simulink model "gtm_aeromodel"  (Simulink 7.2)
settings: Solver=ode45  StartTime=0.0  StopTime=10.0  RelTol=1e-3
undefined symbols (not defined in the file or in its folder): A_BLCG, A_BW, A_CW, A_FSCG, A_FSREF_in, A_SW, A_WLCG, A_WLREF, ALPHA0, bclowb, bclowbx_FMACH, bcmowb, bcmowbx_FHP, bcmowby_FMACH, cda, cdax_FLPDEF, cddr, cddrx_FMACH, cdo, cdox_FLPDEF, cdt1, cdt1x_mach, cdt2, cdt2x_mach, cdto, cdtox_mach, cdwb, cdwbx_FALPHA, cdwby_FMACH, clat, clatfr, clatfrx_FHP, clatfry_FMACH, clatx_mach, clawbfr, clawbfrx_FHP, clawbfry_FMACH, cldefr, cldefrx_FHP, cldefry_FMACH, cldtab, cldtabx_FMACH, clqwb, clqwbfr, clqwbfrx_FHP, clqwbfry_FMACH, clqwbx_mach, cltdd, cltddx_FHP, cltddy_FMACH, clwb, clwbtdd, clwbtddx_FHP, clwbtddy_FMACH, clwbx_FALPHA, clwby_FMACH, clwbzdd, clwbzddx_FHP, clwbzddy_FMACH, clzdd ... (+196)
libraries: model_lib x1
(part 7 of 10)

== system gtm_aeromodel/get aero forces and moments/AERODYNAMICS/Aero Incidence Angles/DOWNWASH/epswb_plus_alphadot/despoflex ==
  altitude : Inport  OutDataType=sfix(16)  OutScaling=2^0
  Mach : Inport  Port=2  OutDataType=sfix(16)  OutScaling=2^0
  Enable : EnablePort
  Fcn : Fcn  Expr=1/u
  Product : Product  OutDataType=sfix(16)  OutScaling=2^0  SaturateOnIntegerOverflow=on  RndMeth=Zero  InputSameDT=on  OutDataTypeStr=Inherit: Same as first input
  clatfr : Subsystem  mask(2-D Table){y=clatfrx_FHP, z=clatfry_FMACH, tab=clatfr}
      mask prompts: y "Y vector:"; z "Z vector:"; tab "Table:"
      mask help: 2-D Table Look Up. Enter monotonic Y and Z vectors and a matrix of 2-D tables. See the help for more info.
      mask Help: The Y and Z vectors must be monotonic.  Y  indexes into the columns of the 2-D table & Z indexes into the rows of the 2-D tables.   The input values are y and z respectively (e.g., top port = y).
      mask Display: plot(-10,-10,110,110,[90,50,10],[90,40,30],[90,50,10],[50,26,20],[90,50,10],[22,13,10])
  cmatfr : Subsystem  mask(2-D Table){y=cmatfrx_FHP, z=cmatfry_FMACH, tab=cmatfr}
      mask prompts: y "Y vector:"; z "Z vector:"; tab "Table:"
      mask help: 2-D Table Look Up. Enter monotonic Y and Z vectors and a matrix of 2-D tables. See the help for more info.
      mask Help: The Y and Z vectors must be monotonic.  Y  indexes into the columns of the 2-D table & Z indexes into the rows of the 2-D tables.   The input values are y and z respectively (e.g., top port = y).
      mask Display: plot(-10,-10,110,110,[90,50,10],[90,40,30],[90,50,10],[50,26,20],[90,50,10],[22,13,10])
  depsoflex : Subsystem  mask(2-D Table){y=depsoflexx_FHP, z=depsoflexy_FMACH, tab=depsoflex}
      mask prompts: y "Y vector:"; z "Z vector:"; tab "Table:"
      mask help: 2-D Table Look Up. Enter monotonic Y and Z vectors and a matrix of 2-D tables. See the help for more info.
      mask Help: The Y and Z vectors must be monotonic.  Y  indexes into the columns of the 2-D table & Z indexes into the rows of the 2-D tables.   The input values are y and z respectively (e.g., top port = y).
      mask Display: plot(-10,-10,110,110,[90,50,10],[90,40,30],[90,50,10],[50,26,20],[90,50,10],[22,13,10])
  epsafr_ : Subsystem  mask(2-D Table){y=epsafrx_FHP, z=epsafry_FMACH, tab=epsafr}
      mask prompts: y "Y vector:"; z "Z vector:"; tab "Table:"
      mask help: 2-D Table Look Up. Enter monotonic Y and Z vectors and a matrix of 2-D tables. See the help for more info.
      mask Help: The Y and Z vectors must be monotonic.  Y  indexes into the columns of the 2-D table & Z indexes into the rows of the 2-D tables.   The input values are y and z respectively (e.g., top port = y).
      mask Display: plot(-10,-10,110,110,[90,50,10],[90,40,30],[90,50,10],[50,26,20],[90,50,10],[22,13,10])
  r2d : Gain  Gain=constants.r2d  ParameterDataType=sfix(16)  ParameterScaling=2^0  OutDataType=sfix(16)  OutScaling=2^0  SaturateOnIntegerOverflow=on  OutDataTypeStr=Inherit: Same as input  ParamDataTypeStr=Inherit: Same as input
  epsafr : Outport  OutDataType=sfix(16)  OutScaling=2^0  InitialOutput=0
  cmocl_atr : Outport  Port=2  OutDataType=sfix(16)  OutScaling=2^0  InitialOutput=0
  despoflex : Outport  Port=3  OutDataType=sfix(16)  OutScaling=2^0  InitialOutput=0
  wires:
  Product/1 -> cmocl_atr/1
  Fcn/1 -> Product/2
  cmatfr/1(Interp Value) -> Product/1
  clatfr/1(Interp Value) -> Fcn/1
  epsafr_/1(Interp Value) -> epsafr/1
  Mach/1 -> clatfr/2(Z), cmatfr/2(Z), epsafr_/2(Z), depsoflex/2(Z)
  altitude/1 -> clatfr/1(Y), cmatfr/1(Y), epsafr_/1(Y), depsoflex/1(Y)
  depsoflex/1(Interp Value) -> r2d/1
  r2d/1 -> despoflex/1

== system gtm_aeromodel/get aero forces and moments/AERODYNAMICS/Aero Incidence Angles/DOWNWASH/epswb_plus_alphadot/epsa ==
  Z : Inport  OutDataType=sfix(16)  OutScaling=2^0
  S-Function : S-Function  FunctionName=table1v5  Parameters=z,tab  EnableBusSupport=off
  Interp Value : Outport  OutDataType=sfix(16)  OutScaling=2^0
  wires:
  Z/1 -> S-Function/1
  S-Function/1 -> Interp Value/1

== system gtm_aeromodel/get aero forces and moments/AERODYNAMICS/Aero Incidence Angles/DOWNWASH/epswb_plus_alphadot/epsodsb ==
  Y : Inport  OutDataType=sfix(16)  OutScaling=2^0
  Z : Inport  Port=2  OutDataType=sfix(16)  OutScaling=2^0
  Mux : Mux  Inputs=2
  S-Function : S-Function  FunctionName=table2v5  Parameters=y,z,tab  EnableBusSupport=off
  Interp Value : Outport  OutDataType=sfix(16)  OutScaling=2^0
  wires:
  Mux/1 -> S-Function/1
  S-Function/1 -> Interp Value/1
  Y/1 -> Mux/1
  Z/1 -> Mux/2

== system gtm_aeromodel/get aero forces and moments/AERODYNAMICS/Aero Incidence Angles/DOWNWASH/sb_df_int/epsdsbdf_ ==
  X : Inport  OutDataType=sfix(16)  OutScaling=2^0
  Y : Inport  Port=2  OutDataType=sfix(16)  OutScaling=2^0
  Z : Inport  Port=3  OutDataType=sfix(16)  OutScaling=2^0
  Mux : Mux  Inputs=3
  S-Function : S-Function  FunctionName=table3v5  Parameters=x,y,z,tab  EnableBusSupport=off
  Interp Value : Outport  OutDataType=sfix(16)  OutScaling=2^0
  wires:
  Z/1 -> Mux/3
  Y/1 -> Mux/2
  X/1 -> Mux/1
  Mux/1 -> S-Function/1
  S-Function/1 -> Interp Value/1

== system gtm_aeromodel/get aero forces and moments/AERODYNAMICS/Aero Incidence Angles/DOWNWASH/sb_df_int/epsdsbdf_1 ==
  X : Inport  OutDataType=sfix(16)  OutScaling=2^0
  Y : Inport  Port=2  OutDataType=sfix(16)  OutScaling=2^0
  Z : Inport  Port=3  OutDataType=sfix(16)  OutScaling=2^0
  Mux : Mux  Inputs=3
  S-Function : S-Function  FunctionName=table3v5  Parameters=x,y,z,tab  EnableBusSupport=off
  Interp Value : Outport  OutDataType=sfix(16)  OutScaling=2^0
  wires:
  S-Function/1 -> Interp Value/1
  Mux/1 -> S-Function/1
  X/1 -> Mux/1
  Y/1 -> Mux/2
  Z/1 -> Mux/3

== system gtm_aeromodel/get aero forces and moments/AERODYNAMICS/Aero Incidence Angles/DOWNWASH/sb_df_int/epsodsb ==
  Y : Inport  OutDataType=sfix(16)  OutScaling=2^0
  Z : Inport  Port=2  OutDataType=sfix(16)  OutScaling=2^0
  Mux : Mux  Inputs=2
  S-Function : S-Function  FunctionName=table2v5  Parameters=y,z,tab  EnableBusSupport=off
  Interp Value : Outport  OutDataType=sfix(16)  OutScaling=2^0
  wires:
  Z/1 -> Mux/2
  Y/1 -> Mux/1
  S-Function/1 -> Interp Value/1
  Mux/1 -> S-Function/1

== system gtm_aeromodel/get aero forces and moments/AERODYNAMICS/Aero Incidence Angles/DOWNWASH/sb_df_int/epsodsb1 ==
  Y : Inport  OutDataType=sfix(16)  OutScaling=2^0
  Z : Inport  Port=2  OutDataType=sfix(16)  OutScaling=2^0
  Mux : Mux  Inputs=2
  S-Function : S-Function  FunctionName=table2v5  Parameters=y,z,tab  EnableBusSupport=off
  Interp Value : Outport  OutDataType=sfix(16)  OutScaling=2^0
  wires:
  Mux/1 -> S-Function/1
  S-Function/1 -> Interp Value/1
  Y/1 -> Mux/1
  Z/1 -> Mux/2

== system gtm_aeromodel/get aero forces and moments/AERODYNAMICS/Aero Incidence Angles/DOWNWASH/sp_int/epsdsldf ==
  X : Inport  OutDataType=sfix(16)  OutScaling=2^0
  Y : Inport  Port=2  OutDataType=sfix(16)  OutScaling=2^0
  Z : Inport  Port=3  OutDataType=sfix(16)  OutScaling=2^0
  Mux : Mux  Inputs=3
  S-Function : S-Function  FunctionName=table3v5  Parameters=x,y,z,tab  EnableBusSupport=off
  Interp Value : Outport  OutDataType=sfix(16)  OutScaling=2^0
  wires:
  Z/1 -> Mux/3
  Y/1 -> Mux/2
  X/1 -> Mux/1
  Mux/1 -> S-Function/1
  S-Function/1 -> Interp Value/1

== system gtm_aeromodel/get aero forces and moments/AERODYNAMICS/Aero Incidence Angles/DOWNWASH/sp_int/epsdsldf1 ==
  X : Inport  OutDataType=sfix(16)  OutScaling=2^0
  Y : Inport  Port=2  OutDataType=sfix(16)  OutScaling=2^0
  Z : Inport  Port=3  OutDataType=sfix(16)  OutScaling=2^0
  Mux : Mux  Inputs=3
  S-Function : S-Function  FunctionName=table3v5  Parameters=x,y,z,tab  EnableBusSupport=off
  Interp Value : Outport  OutDataType=sfix(16)  OutScaling=2^0
  wires:
  S-Function/1 -> Interp Value/1
  Mux/1 -> S-Function/1
  X/1 -> Mux/1
  Y/1 -> Mux/2
  Z/1 -> Mux/3

== system gtm_aeromodel/get aero forces and moments/AERODYNAMICS/Aero Incidence Angles/DOWNWASH/sp_int/epsdsldf2 ==
  X : Inport  OutDataType=sfix(16)  OutScaling=2^0
  Y : Inport  Port=2  OutDataType=sfix(16)  OutScaling=2^0
  Z : Inport  Port=3  OutDataType=sfix(16)  OutScaling=2^0
  Mux : Mux  Inputs=3
  S-Function : S-Function  FunctionName=table3v5  Parameters=x,y,z,tab  EnableBusSupport=off
  Interp Value : Outport  OutDataType=sfix(16)  OutScaling=2^0
  wires:
  Z/1 -> Mux/3
  Y/1 -> Mux/2
  X/1 -> Mux/1
  Mux/1 -> S-Function/1
  S-Function/1 -> Interp Value/1

== system gtm_aeromodel/get aero forces and moments/AERODYNAMICS/Aero Incidence Angles/DOWNWASH/sp_int/epsodsl ==
  Y : Inport  OutDataType=sfix(16)  OutScaling=2^0
  Z : Inport  Port=2  OutDataType=sfix(16)  OutScaling=2^0
  Mux : Mux  Inputs=2
  S-Function : S-Function  FunctionName=table2v5  Parameters=y,z,tab  EnableBusSupport=off
  Interp Value : Outport  OutDataType=sfix(16)  OutScaling=2^0
  wires:
  Z/1 -> Mux/2
  Y/1 -> Mux/1
  S-Function/1 -> Interp Value/1
  Mux/1 -> S-Function/1

== system gtm_aeromodel/get aero forces and moments/AERODYNAMICS/Aero Incidence Angles/DOWNWASH/sp_int/epsodsl1 ==
  Y : Inport  OutDataType=sfix(16)  OutScaling=2^0
  Z : Inport  Port=2  OutDataType=sfix(16)  OutScaling=2^0
  Mux : Mux  Inputs=2
  S-Function : S-Function  FunctionName=table2v5  Parameters=y,z,tab  EnableBusSupport=off
  Interp Value : Outport  OutDataType=sfix(16)  OutScaling=2^0
  wires:
  Mux/1 -> S-Function/1
  S-Function/1 -> Interp Value/1
  Y/1 -> Mux/1
  Z/1 -> Mux/2

== system gtm_aeromodel/get aero forces and moments/AERODYNAMICS/Aero Incidence Angles/DOWNWASH/sp_int/epsodsl2 ==
  Y : Inport  OutDataType=sfix(16)  OutScaling=2^0
  Z : Inport  Port=2  OutDataType=sfix(16)  OutScaling=2^0
  Mux : Mux  Inputs=2
  S-Function : S-Function  FunctionName=table2v5  Parameters=y,z,tab  EnableBusSupport=off
  Interp Value : Outport  OutDataType=sfix(16)  OutScaling=2^0
  wires:
  Mux/1 -> S-Function/1
  S-Function/1 -> Interp Value/1
  Y/1 -> Mux/1
  Z/1 -> Mux/2

== system gtm_aeromodel/get aero forces and moments/AERODYNAMICS/Aero Incidence Angles/TAIL ANGLES/dalphat_flex/clat_ ==
  Z : Inport  OutDataType=sfix(16)  OutScaling=2^0
  S-Function : S-Function  FunctionName=table1v5  Parameters=z,tab  EnableBusSupport=off
  Interp Value : Outport  OutDataType=sfix(16)  OutScaling=2^0
  wires:
  S-Function/1 -> Interp Value/1
  Z/1 -> S-Function/1

== system gtm_aeromodel/get aero forces and moments/AERODYNAMICS/Aero Incidence Angles/TAIL ANGLES/dalphat_flex/clatfr ==
  Y : Inport  OutDataType=sfix(16)  OutScaling=2^0
  Z : Inport  Port=2  OutDataType=sfix(16)  OutScaling=2^0
  Mux : Mux  Inputs=2
  S-Function : S-Function  FunctionName=table2v5  Parameters=y,z,tab  EnableBusSupport=off
  Interp Value : Outport  OutDataType=sfix(16)  OutScaling=2^0
  wires:
  Mux/1 -> S-Function/1
  S-Function/1 -> Interp Value/1
  Y/1 -> Mux/1
  Z/1 -> Mux/2

== system gtm_aeromodel/get aero forces and moments/AERODYNAMICS/Aero Incidence Angles/TAIL ANGLES/dalphat_flex/cldefr ==
  Y : Inport  OutDataType=sfix(16)  OutScaling=2^0
  Z : Inport  Port=2  OutDataType=sfix(16)  OutScaling=2^0
  Mux : Mux  Inputs=2
  S-Function : S-Function  FunctionName=table2v5  Parameters=y,z,tab  EnableBusSupport=off
  Interp Value : Outport  OutDataType=sfix(16)  OutScaling=2^0
  wires:
  Mux/1 -> S-Function/1
  S-Function/1 -> Interp Value/1
  Y/1 -> Mux/1
  Z/1 -> Mux/2

== system gtm_aeromodel/get aero forces and moments/AERODYNAMICS/Aero Incidence Angles/TAIL ANGLES/dalphat_flex/cldetab ==
  Z : Inport  OutDataType=sfix(16)  OutScaling=2^0
  S-Function : S-Function  FunctionName=table1v5  Parameters=z,tab  EnableBusSupport=off
  Interp Value : Outport  OutDataType=sfix(16)  OutScaling=2^0
  wires:
  Z/1 -> S-Function/1
  S-Function/1 -> Interp Value/1

== system gtm_aeromodel/get aero forces and moments/AERODYNAMICS/Aero Incidence Angles/TAIL ANGLES/dalphat_flex/dclde ==
  X : Inport  OutDataType=sfix(16)  OutScaling=2^0
  Y : Inport  Port=2  OutDataType=sfix(16)  OutScaling=2^0
  Z : Inport  Port=3  OutDataType=sfix(16)  OutScaling=2^0
  Mux : Mux  Inputs=3
  S-Function : S-Function  FunctionName=table3v5  Parameters=x,y,z,tab  EnableBusSupport=off
  Interp Value : Outport  OutDataType=sfix(16)  OutScaling=2^0
  wires:
  S-Function/1 -> Interp Value/1
  Mux/1 -> S-Function/1
  X/1 -> Mux/1
  Y/1 -> Mux/2
  Z/1 -> Mux/3

== system gtm_aeromodel/get aero forces and moments/AERODYNAMICS/Aero Incidence Angles/TAIL ANGLES/dbetat_flex/cybfr ==
  Y : Inport  OutDataType=sfix(16)  OutScaling=2^0
  Z : Inport  Port=2  OutDataType=sfix(16)  OutScaling=2^0
  Mux : Mux  Inputs=2
  S-Function : S-Function  FunctionName=table2v5  Parameters=y,z,tab  EnableBusSupport=off
  Interp Value : Outport  OutDataType=sfix(16)  OutScaling=2^0
  wires:
  Z/1 -> Mux/2
  Y/1 -> Mux/1
  S-Function/1 -> Interp Value/1
  Mux/1 -> S-Function/1

== system gtm_aeromodel/get aero forces and moments/AERODYNAMICS/Aero Incidence Angles/TAIL ANGLES/dbetat_flex/cybvt ==
  Y : Inport  OutDataType=sfix(16)  OutScaling=2^0
  Z : Inport  Port=2  OutDataType=sfix(16)  OutScaling=2^0
  Mux : Mux  Inputs=2
  S-Function : S-Function  FunctionName=table2v5  Parameters=y,z,tab  EnableBusSupport=off
  Interp Value : Outport  OutDataType=sfix(16)  OutScaling=2^0
  wires:
  Z/1 -> Mux/2
  Y/1 -> Mux/1
  S-Function/1 -> Interp Value/1
  Mux/1 -> S-Function/1

== system gtm_aeromodel/get aero forces and moments/AERODYNAMICS/Aero Incidence Angles/TAIL ANGLES/dbetat_flex/cydr ==
  Z : Inport  OutDataType=sfix(16)  OutScaling=2^0
  S-Function : S-Function  FunctionName=table1v5  Parameters=z,tab  EnableBusSupport=off
  Interp Value : Outport  OutDataType=sfix(16)  OutScaling=2^0
  wires:
  S-Function/1 -> Interp Value/1
  Z/1 -> S-Function/1

== system gtm_aeromodel/get aero forces and moments/AERODYNAMICS/Aero Incidence Angles/TAIL ANGLES/dbetat_flex/cydrfr ==
  Y : Inport  OutDataType=sfix(16)  OutScaling=2^0
  Z : Inport  Port=2  OutDataType=sfix(16)  OutScaling=2^0
  Mux : Mux  Inputs=2
  S-Function : S-Function  FunctionName=table2v5  Parameters=y,z,tab  EnableBusSupport=off
  Interp Value : Outport  OutDataType=sfix(16)  OutScaling=2^0
  wires:
  Z/1 -> Mux/2
  Y/1 -> Mux/1
  S-Function/1 -> Interp Value/1
  Mux/1 -> S-Function/1

== system gtm_aeromodel/get aero forces and moments/AERODYNAMICS/Force  Coefficients/DRAG /CDAIL/dcdda ==
  Z : Inport  OutDataType=sfix(16)  OutScaling=2^0
  S-Function : S-Function  FunctionName=table1v5  Parameters=z,tab  EnableBusSupport=off
  Interp Value : Outport  OutDataType=sfix(16)  OutScaling=2^0
  wires:
  Z/1 -> S-Function/1
  S-Function/1 -> Interp Value/1

== system gtm_aeromodel/get aero forces and moments/AERODYNAMICS/Force  Coefficients/DRAG /CDAIL/dcdda1 ==
  Z : Inport  OutDataType=sfix(16)  OutScaling=2^0
  S-Function : S-Function  FunctionName=table1v5  Parameters=z,tab  EnableBusSupport=off
  Interp Value : Outport  OutDataType=sfix(16)  OutScaling=2^0
  wires:
  S-Function/1 -> Interp Value/1
  Z/1 -> S-Function/1

== system gtm_aeromodel/get aero forces and moments/AERODYNAMICS/Force  Coefficients/DRAG /CDGE/dcdhob ==
  X : Inport  OutDataType=sfix(16)  OutScaling=2^0
  Y : Inport  Port=2  OutDataType=sfix(16)  OutScaling=2^0
  Z : Inport  Port=3  OutDataType=sfix(16)  OutScaling=2^0
  Mux : Mux  Inputs=3
  S-Function : S-Function  FunctionName=table3v5  Parameters=x,y,z,tab  EnableBusSupport=off
  Interp Value : Outport  OutDataType=sfix(16)  OutScaling=2^0
  wires:
  Z/1 -> Mux/3
  Y/1 -> Mux/2
  X/1 -> Mux/1
  Mux/1 -> S-Function/1
  S-Function/1 -> Interp Value/1

== system gtm_aeromodel/get aero forces and moments/AERODYNAMICS/Force  Coefficients/DRAG /CDGEAR/cda ==
  Z : Inport  OutDataType=sfix(16)  OutScaling=2^0
  S-Function : S-Function  FunctionName=table1v5  Parameters=z,tab  EnableBusSupport=off
  Interp Value : Outport  OutDataType=sfix(16)  OutScaling=2^0
  wires:
  Z/1 -> S-Function/1
  S-Function/1 -> Interp Value/1

== system gtm_aeromodel/get aero forces and moments/AERODYNAMICS/Force  Coefficients/DRAG /CDGEAR/cdo ==
  Z : Inport  OutDataType=sfix(16)  OutScaling=2^0
  S-Function : S-Function  FunctionName=table1v5  Parameters=z,tab  EnableBusSupport=off
  Interp Value : Outport  OutDataType=sfix(16)  OutScaling=2^0
  wires:
  Z/1 -> S-Function/1
  S-Function/1 -> Interp Value/1

== system gtm_aeromodel/get aero forces and moments/AERODYNAMICS/Force  Coefficients/DRAG /CDR/cddr ==
  Z : Inport  OutDataType=sfix(16)  OutScaling=2^0
  S-Function : S-Function  FunctionName=table1v5  Parameters=z,tab  EnableBusSupport=off
  Interp Value : Outport  OutDataType=sfix(16)  OutScaling=2^0
  wires:
  Z/1 -> S-Function/1
  S-Function/1 -> Interp Value/1

== system gtm_aeromodel/get aero forces and moments/AERODYNAMICS/Force  Coefficients/DRAG /CDSPOIL/cd_sp_int ==
  flap : Inport  OutDataType=sfix(16)  OutScaling=2^0
  alpha : Inport  Port=2  OutDataType=sfix(16)  OutScaling=2^0
  dsl : Inport  Port=3  OutDataType=sfix(16)  OutScaling=2^0
  dsb : Inport  Port=4  OutDataType=sfix(16)  OutScaling=2^0
  dsr : Inport  Port=5  OutDataType=sfix(16)  OutScaling=2^0
  Enable : EnablePort
  Sum : Sum  Inputs=+-  OutDataType=sfix(16)  OutScaling=2^0  SaturateOnIntegerOverflow=on  InputSameDT=on  OutDataTypeStr=Inherit: Same as first input
  Sum1 : Sum  Inputs=-+  OutDataType=sfix(16)  OutScaling=2^0  SaturateOnIntegerOverflow=on  InputSameDT=on  OutDataTypeStr=Inherit: Same as first input
  Sum2 : Sum  OutDataType=sfix(16)  OutScaling=2^0  SaturateOnIntegerOverflow=on  InputSameDT=on  OutDataTypeStr=Inherit: Same as first input
  dcdwbdsbp : Subsystem  mask(1-2-3 Table){@1=dcdwbdsldfx_DSL, @2=dcdwbdsldfy_FALPHA, @3=dcdwbdsldfz_FLPDEF, @4=dcdwbdsldf}
      mask prompts: @1 "X vector:"; @2 "Y vector:"; @3 "Z vector:"; @4 "Table:"
      mask help: 3-D Table Look Up. Enter monotonic X, Y and Z vectors and a matrix of 2-D tables. See the help for more info.
      mask init:
      | x=@1;y=@2;z=@3;tab=@4;
      mask Help: The X, Y and Z vectors must be monotonic.   The 3-D table is a horizontal concatenation of  2-D tables.  X  indexes into the columns of the 2-D tables & Y indexes into the rows of the 2-D tables.  Z indexes into the table levels (starting with the 1st 2-D table).   The input values are x, y and z respectively (e.g., top port = x).
      mask Display: plot([0 2 2 0 0],[0 0 2 2 0],[0 2 2.9 0.95 0],[2 2 2.7 2.7 2],[2 2.9 2.9 2 2],[0 0.85 2.7 2 0])
  dcdwbdsldf : Subsystem  mask(1-2-3 Table){@1=dcdwbdsldfx_DSL, @2=dcdwbdsldfy_FALPHA, @3=dcdwbdsldfz_FLPDEF, @4=dcdwbdsldf}
      mask prompts: @1 "X vector:"; @2 "Y vector:"; @3 "Z vector:"; @4 "Table:"
      mask help: 3-D Table Look Up. Enter monotonic X, Y and Z vectors and a matrix of 2-D tables. See the help for more info.
      mask init:
      | x=@1;y=@2;z=@3;tab=@4;
      mask Help: The X, Y and Z vectors must be monotonic.   The 3-D table is a horizontal concatenation of  2-D tables.  X  indexes into the columns of the 2-D tables & Y indexes into the rows of the 2-D tables.  Z indexes into the table levels (starting with the 1st 2-D table).   The input values are x, y and z respectively (e.g., top port = x).
      mask Display: plot([0 2 2 0 0],[0 0 2 2 0],[0 2 2.9 0.95 0],[2 2 2.7 2.7 2],[2 2.9 2.9 2 2],[0 0.85 2.7 2 0])
  dcdwbdsldf1 : Subsystem  mask(1-2-3 Table){@1=dcdwbdsldfx_DSL, @2=dcdwbdsldfy_FALPHA, @3=dcdwbdsldfz_FLPDEF, @4=dcdwbdsldf}
      mask prompts: @1 "X vector:"; @2 "Y vector:"; @3 "Z vector:"; @4 "Table:"
      mask help: 3-D Table Look Up. Enter monotonic X, Y and Z vectors and a matrix of 2-D tables. See the help for more info.
      mask init:
      | x=@1;y=@2;z=@3;tab=@4;
      mask Help: The X, Y and Z vectors must be monotonic.   The 3-D table is a horizontal concatenation of  2-D tables.  X  indexes into the columns of the 2-D tables & Y indexes into the rows of the 2-D tables.  Z indexes into the table levels (starting with the 1st 2-D table).   The input values are x, y and z respectively (e.g., top port = x).
      mask Display: plot([0 2 2 0 0],[0 0 2 2 0],[0 2 2.9 0.95 0],[2 2 2.7 2.7 2],[2 2.9 2.9 2 2],[0 0.85 2.7 2 0])
  cd_sp_int : Outport  OutDataType=sfix(16)  OutScaling=2^0  InitialOutput=0
  wires:
  Sum1/1 -> Sum2/2
  Sum/1 -> Sum2/1
  Sum2/1 -> cd_sp_int/1
  dcdwbdsbp/1(Interp Value) -> Sum1/1, Sum/2
  dcdwbdsldf1/1(Interp Value) -> Sum1/2
  flap/1 -> dcdwbdsldf/3(Z), dcdwbdsbp/3(Z), dcdwbdsldf1/3(Z)
  dcdwbdsldf/1(Interp Value) -> Sum/1
  alpha/1 -> dcdwbdsldf/2(Y), dcdwbdsbp/2(Y), dcdwbdsldf1/2(Y)
  dsl/1 -> dcdwbdsldf/1(X)
  dsr/1 -> dcdwbdsldf1/1(X)
  dsb/1 -> dcdwbdsbp/1(X)

== system gtm_aeromodel/get aero forces and moments/AERODYNAMICS/Force  Coefficients/DRAG /CDSPOIL/dcdwbdsb ==
  X : Inport  OutDataType=sfix(16)  OutScaling=2^0
  Y : Inport  Port=2  OutDataType=sfix(16)  OutScaling=2^0
  Z : Inport  Port=3  OutDataType=sfix(16)  OutScaling=2^0
  Mux : Mux  Inputs=3
  S-Function : S-Function  FunctionName=table3v5  Parameters=x,y,z,tab  EnableBusSupport=off
  Interp Value : Outport  OutDataType=sfix(16)  OutScaling=2^0
  wires:
  Z/1 -> Mux/3
  Y/1 -> Mux/2
  X/1 -> Mux/1
  Mux/1 -> S-Function/1
  S-Function/1 -> Interp Value/1

== system gtm_aeromodel/get aero forces and moments/AERODYNAMICS/Force  Coefficients/DRAG /CDSPOIL/dcdwbdsb_ ==
  X : Inport  OutDataType=sfix(16)  OutScaling=2^0
  Y : Inport  Port=2  OutDataType=sfix(16)  OutScaling=2^0
  Z : Inport  Port=3  OutDataType=sfix(16)  OutScaling=2^0
  Mux : Mux  Inputs=3
  S-Function : S-Function  FunctionName=table3v5  Parameters=x,y,z,tab  EnableBusSupport=off
  Interp Value : Outport  OutDataType=sfix(16)  OutScaling=2^0
  wires:
  S-Function/1 -> Interp Value/1
  Mux/1 -> S-Function/1
  X/1 -> Mux/1
  Y/1 -> Mux/2
  Z/1 -> Mux/3

== system gtm_aeromodel/get aero forces and moments/AERODYNAMICS/Force  Coefficients/DRAG /CDSPOIL/dcdwbdsl ==
  X : Inport  OutDataType=sfix(16)  OutScaling=2^0
  Y : Inport  Port=2  OutDataType=sfix(16)  OutScaling=2^0
  Z : Inport  Port=3  OutDataType=sfix(16)  OutScaling=2^0
  Mux : Mux  Inputs=3
  S-Function : S-Function  FunctionName=table3v5  Parameters=x,y,z,tab  EnableBusSupport=off
  Interp Value : Outport  OutDataType=sfix(16)  OutScaling=2^0
  wires:
  Z/1 -> Mux/3
  Y/1 -> Mux/2
  X/1 -> Mux/1
  Mux/1 -> S-Function/1
  S-Function/1 -> Interp Value/1

== system gtm_aeromodel/get aero forces and moments/AERODYNAMICS/Force  Coefficients/DRAG /CDSPOIL/dcdwbdsl1 ==
  X : Inport  OutDataType=sfix(16)  OutScaling=2^0
  Y : Inport  Port=2  OutDataType=sfix(16)  OutScaling=2^0
  Z : Inport  Port=3  OutDataType=sfix(16)  OutScaling=2^0
  Mux : Mux  Inputs=3
  S-Function : S-Function  FunctionName=table3v5  Parameters=x,y,z,tab  EnableBusSupport=off
  Interp Value : Outport  OutDataType=sfix(16)  OutScaling=2^0
  wires:
  S-Function/1 -> Interp Value/1
  Mux/1 -> S-Function/1
  X/1 -> Mux/1
  Y/1 -> Mux/2
  Z/1 -> Mux/3

== system gtm_aeromodel/get aero forces and moments/AERODYNAMICS/Force  Coefficients/DRAG /CDSPOIL/dcdwbdsl_ ==
  X : Inport  OutDataType=sfix(16)  OutScaling=2^0
  Y : Inport  Port=2  OutDataType=sfix(16)  OutScaling=2^0
  Z : Inport  Port=3  OutDataType=sfix(16)  OutScaling=2^0
  Mux : Mux  Inputs=3
  S-Function : S-Function  FunctionName=table3v5  Parameters=x,y,z,tab  EnableBusSupport=off
  Interp Value : Outport  OutDataType=sfix(16)  OutScaling=2^0
  wires:
  S-Function/1 -> Interp Value/1
  Mux/1 -> S-Function/1
  X/1 -> Mux/1
  Y/1 -> Mux/2
  Z/1 -> Mux/3

== system gtm_aeromodel/get aero forces and moments/AERODYNAMICS/Force  Coefficients/DRAG /CDSPOIL/dcdwbdsl_1 ==
  X : Inport  OutDataType=sfix(16)  OutScaling=2^0
  Y : Inport  Port=2  OutDataType=sfix(16)  OutScaling=2^0
  Z : Inport  Port=3  OutDataType=sfix(16)  OutScaling=2^0
  Mux : Mux  Inputs=3
  S-Function : S-Function  FunctionName=table3v5  Parameters=x,y,z,tab  EnableBusSupport=off
  Interp Value : Outport  OutDataType=sfix(16)  OutScaling=2^0
  wires:
  Z/1 -> Mux/3
  Y/1 -> Mux/2
  X/1 -> Mux/1
  Mux/1 -> S-Function/1
  S-Function/1 -> Interp Value/1

== system gtm_aeromodel/get aero forces and moments/AERODYNAMICS/Force  Coefficients/DRAG /CDSPOIL/dcdwbdsl_2 ==
  X : Inport  OutDataType=sfix(16)  OutScaling=2^0
  Y : Inport  Port=2  OutDataType=sfix(16)  OutScaling=2^0
  Z : Inport  Port=3  OutDataType=sfix(16)  OutScaling=2^0
  Mux : Mux  Inputs=3
  S-Function : S-Function  FunctionName=table3v5  Parameters=x,y,z,tab  EnableBusSupport=off
  Interp Value : Outport  OutDataType=sfix(16)  OutScaling=2^0
  wires:
  S-Function/1 -> Interp Value/1
  Mux/1 -> S-Function/1
  X/1 -> Mux/1
  Y/1 -> Mux/2
  Z/1 -> Mux/3

== system gtm_aeromodel/get aero forces and moments/AERODYNAMICS/Force  Coefficients/DRAG /CDSPOIL/dcdwbdsl_3 ==
  X : Inport  OutDataType=sfix(16)  OutScaling=2^0
  Y : Inport  Port=2  OutDataType=sfix(16)  OutScaling=2^0
  Z : Inport  Port=3  OutDataType=sfix(16)  OutScaling=2^0
  Mux : Mux  Inputs=3
  S-Function : S-Function  FunctionName=table3v5  Parameters=x,y,z,tab  EnableBusSupport=off
  Interp Value : Outport  OutDataType=sfix(16)  OutScaling=2^0
  wires:
  Z/1 -> Mux/3
  Y/1 -> Mux/2
  X/1 -> Mux/1
  Mux/1 -> S-Function/1
  S-Function/1 -> Interp Value/1

== system gtm_aeromodel/get aero forces and moments/AERODYNAMICS/Force  Coefficients/DRAG /CDTP/cdt1 ==
  Z : Inport  OutDataType=sfix(16)  OutScaling=2^0
  S-Function : S-Function  FunctionName=table1v5  Parameters=z,tab  EnableBusSupport=off
  Interp Value : Outport  OutDataType=sfix(16)  OutScaling=2^0
  wires:
  Z/1 -> S-Function/1
  S-Function/1 -> Interp Value/1

== system gtm_aeromodel/get aero forces and moments/AERODYNAMICS/Force  Coefficients/DRAG /CDTP/cdt2 ==
  Z : Inport  OutDataType=sfix(16)  OutScaling=2^0
  S-Function : S-Function  FunctionName=table1v5  Parameters=z,tab  EnableBusSupport=off
  Interp Value : Outport  OutDataType=sfix(16)  OutScaling=2^0
  wires:
  Z/1 -> S-Function/1
  S-Function/1 -> Interp Value/1

== system gtm_aeromodel/get aero forces and moments/AERODYNAMICS/Force  Coefficients/DRAG /CDTP/cdto ==
  Z : Inport  OutDataType=sfix(16)  OutScaling=2^0
  S-Function : S-Function  FunctionName=table1v5  Parameters=z,tab  EnableBusSupport=off
  Interp Value : Outport  OutDataType=sfix(16)  OutScaling=2^0
  wires:
  Z/1 -> S-Function/1
  S-Function/1 -> Interp Value/1

== system gtm_aeromodel/get aero forces and moments/AERODYNAMICS/Force  Coefficients/DRAG /CDWB/CDWBFLEX ==
  alpha : Inport  OutDataType=sfix(16)  OutScaling=2^0
  Mach : Inport  Port=2  OutDataType=sfix(16)  OutScaling=2^0
  altitude : Inport  Port=3  OutDataType=sfix(16)  OutScaling=2^0
  Enable : EnablePort
  dcdflex_ : Subsystem  mask(1-2-3 Table){@1=dcdflexx_FALPHA, @2=dcdflexy_FMACH, @3=dcdflexz_FHP, @4=dcdflex}
      mask prompts: @1 "X vector:"; @2 "Y vector:"; @3 "Z vector:"; @4 "Table:"
      mask help: 3-D Table Look Up. Enter monotonic X, Y and Z vectors and a matrix of 2-D tables. See the help for more info.
      mask init:
      | x=@1;y=@2;z=@3;tab=@4;
      mask Help: The X, Y and Z vectors must be monotonic.   The 3-D table is a horizontal concatenation of  2-D tables.  X  indexes into the columns of the 2-D tables & Y indexes into the rows of the 2-D tables.  Z indexes into the table levels (starting with the 1st 2-D table).   The input values are x, y and z respectively (e.g., top port = x).
      mask Display: plot([0 2 2 0 0],[0 0 2 2 0],[0 2 2.9 0.95 0],[2 2 2.7 2.7 2],[2 2.9 2.9 2 2],[0 0.85 2.7 2 0])
  dcdflex : Outport  OutDataType=sfix(16)  OutScaling=2^0  InitialOutput=0
  wires:
  altitude/1 -> dcdflex_/3(Z)
  dcdflex_/1(Interp Value) -> dcdflex/1
  Mach/1 -> dcdflex_/2(Y)
  alpha/1 -> dcdflex_/1(X)

== system gtm_aeromodel/get aero forces and moments/AERODYNAMICS/Force  Coefficients/DRAG /CDWB/cd_flap_ ==
  flap : Inport  OutDataType=sfix(16)  OutScaling=2^0
  alpha : Inport  Port=2  OutDataType=sfix(16)  OutScaling=2^0
  dsb : Inport  Port=3  OutDataType=sfix(16)  OutScaling=2^0
  Enable : EnablePort
  DSB : Constant  Value=0.0  OutDataType=sfix(16)  OutScaling=2^0
  MACH : Constant  Value=0.178  OutDataType=sfix(16)  OutScaling=2^0
  Sum : Sum  Inputs=+-  OutDataType=sfix(16)  OutScaling=2^0  SaturateOnIntegerOverflow=on  InputSameDT=on  OutDataTypeStr=Inherit: Same as first input
  Sum1 : Sum  Inputs=+--  OutDataType=sfix(16)  OutScaling=2^0  SaturateOnIntegerOverflow=on  InputSameDT=on  OutDataTypeStr=Inherit: Same as first input
  cdwb : Subsystem  mask(2-D Table){y=cdwbx_FALPHA, z=cdwby_FMACH, tab=cdwb}
      mask prompts: y "Y vector:"; z "Z vector:"; tab "Table:"
      mask help: 2-D Table Look Up. Enter monotonic Y and Z vectors and a matrix of 2-D tables. See the help for more info.
      mask Help: The Y and Z vectors must be monotonic.  Y  indexes into the columns of the 2-D table & Z indexes into the rows of the 2-D tables.   The input values are y and z respectively (e.g., top port = y).
      mask Display: plot(-10,-10,110,110,[90,50,10],[90,40,30],[90,50,10],[50,26,20],[90,50,10],[22,13,10])
  cdwbdsbdf : Subsystem  mask(1-2-3 Table){@1=cdwbdsbdfx_DSB, @2=cdwbdsbdfy_FALPHA, @3=cdwbdsbdfz_FLPDEF, @4=cdwbdsbdf}
      mask prompts: @1 "X vector:"; @2 "Y vector:"; @3 "Z vector:"; @4 "Table:"
      mask help: 3-D Table Look Up. Enter monotonic X, Y and Z vectors and a matrix of 2-D tables. See the help for more info.
      mask init:
      | x=@1;y=@2;z=@3;tab=@4;
      mask Help: The X, Y and Z vectors must be monotonic.   The 3-D table is a horizontal concatenation of  2-D tables.  X  indexes into the columns of the 2-D tables & Y indexes into the rows of the 2-D tables.  Z indexes into the table levels (starting with the 1st 2-D table).   The input values are x, y and z respectively (e.g., top port = x).
      mask Display: plot([0 2 2 0 0],[0 0 2 2 0],[0 2 2.9 0.95 0],[2 2 2.7 2.7 2],[2 2.9 2.9 2 2],[0 0.85 2.7 2 0])
  cdwbdsbdf1 : Subsystem  mask(1-2-3 Table){@1=cdwbdsbdfx_DSB, @2=cdwbdsbdfy_FALPHA, @3=cdwbdsbdfz_FLPDEF, @4=cdwbdsbdf}
      mask prompts: @1 "X vector:"; @2 "Y vector:"; @3 "Z vector:"; @4 "Table:"
      mask help: 3-D Table Look Up. Enter monotonic X, Y and Z vectors and a matrix of 2-D tables. See the help for more info.
      mask init:
      | x=@1;y=@2;z=@3;tab=@4;
      mask Help: The X, Y and Z vectors must be monotonic.   The 3-D table is a horizontal concatenation of  2-D tables.  X  indexes into the columns of the 2-D tables & Y indexes into the rows of the 2-D tables.  Z indexes into the table levels (starting with the 1st 2-D table).   The input values are x, y and z respectively (e.g., top port = x).
      mask Display: plot([0 2 2 0 0],[0 0 2 2 0],[0 2 2.9 0.95 0],[2 2 2.7 2.7 2],[2 2.9 2.9 2 2],[0 0.85 2.7 2 0])
  dcdwbdsbdf2 : Subsystem  mask(1-2-3 Table){@1=dcdwbdsbx_DSB, @2=dcdwbdsby_ALPHA, @3=dcdwbdsbz_FMACH, @4=dcdwbdsb}
      mask prompts: @1 "X vector:"; @2 "Y vector:"; @3 "Z vector:"; @4 "Table:"
      mask help: 3-D Table Look Up. Enter monotonic X, Y and Z vectors and a matrix of 2-D tables. See the help for more info.
      mask init:
      | x=@1;y=@2;z=@3;tab=@4;
      mask Help: The X, Y and Z vectors must be monotonic.   The 3-D table is a horizontal concatenation of  2-D tables.  X  indexes into the columns of the 2-D tables & Y indexes into the rows of the 2-D tables.  Z indexes into the table levels (starting with the 1st 2-D table).   The input values are x, y and z respectively (e.g., top port = x).
      mask Display: plot([0 2 2 0 0],[0 0 2 2 0],[0 2 2.9 0.95 0],[2 2 2.7 2.7 2],[2 2.9 2.9 2 2],[0 0.85 2.7 2 0])
  cd_flap : Outport  OutDataType=sfix(16)  OutScaling=2^0  InitialOutput=0
  dcdsbfint : Outport  Port=2  OutDataType=sfix(16)  OutScaling=2^0  InitialOutput=0
  wires:
  DSB/1 -> cdwbdsbdf/1(X)
  alpha/1 -> cdwb/1(Y), cdwbdsbdf/2(Y), cdwbdsbdf1/2(Y), dcdwbdsbdf2/2(Y)
  flap/1 -> cdwbdsbdf/3(Z), cdwbdsbdf1/3(Z)
  Sum/1 -> cd_flap/1
  cdwbdsbdf1/1(Interp Value) -> Sum1/1
  cdwbdsbdf/1(Interp Value) -> Sum/1, Sum1/2
  Sum1/1 -> dcdsbfint/1
  MACH/1 -> cdwb/2(Z), dcdwbdsbdf2/3(Z)
  dsb/1 -> cdwbdsbdf1/1(X), dcdwbdsbdf2/1(X)
  dcdwbdsbdf2/1(Interp Value) -> Sum1/3
  cdwb/1(Interp Value) -> Sum/2

== system gtm_aeromodel/get aero forces and moments/AERODYNAMICS/Force  Coefficients/DRAG /CDWB/cdwb_clean ==
  Y : Inport  OutDataType=sfix(16)  OutScaling=2^0
  Z : Inport  Port=2  OutDataType=sfix(16)  OutScaling=2^0
  Mux : Mux  Inputs=2
  S-Function : S-Function  FunctionName=table2v5  Parameters=y,z,tab  EnableBusSupport=off
  Interp Value : Outport  OutDataType=sfix(16)  OutScaling=2^0
  wires:
  Z/1 -> Mux/2
  Y/1 -> Mux/1
  S-Function/1 -> Interp Value/1
  Mux/1 -> S-Function/1

== system gtm_aeromodel/get aero forces and moments/AERODYNAMICS/Force  Coefficients/DRAG /DCDDEL/dcdde_ ==
  X : Inport  OutDataType=sfix(16)  OutScaling=2^0
  Y : Inport  Port=2  OutDataType=sfix(16)  OutScaling=2^0
  Z : Inport  Port=3  OutDataType=sfix(16)  OutScaling=2^0
  Mux : Mux  Inputs=3
  S-Function : S-Function  FunctionName=table3v5  Parameters=x,y,z,tab  EnableBusSupport=off
  Interp Value : Outport  OutDataType=sfix(16)  OutScaling=2^0
  wires:
  S-Function/1 -> Interp Value/1
  Mux/1 -> S-Function/1
  X/1 -> Mux/1
  Y/1 -> Mux/2
  Z/1 -> Mux/3

== system gtm_aeromodel/get aero forces and moments/AERODYNAMICS/Force  Coefficients/LIFT/CLDETAB/cldetab_ ==
  Z : Inport  OutDataType=sfix(16)  OutScaling=2^0
  S-Function : S-Function  FunctionName=table1v5  Parameters=z,tab  EnableBusSupport=off
  Interp Value : Outport  OutDataType=sfix(16)  OutScaling=2^0
  wires:
  S-Function/1 -> Interp Value/1
  Z/1 -> S-Function/1

== system gtm_aeromodel/get aero forces and moments/AERODYNAMICS/Force  Coefficients/LIFT/CLGE/dclhob ==
  X : Inport  OutDataType=sfix(16)  OutScaling=2^0
  Y : Inport  Port=2  OutDataType=sfix(16)  OutScaling=2^0
  Z : Inport  Port=3  OutDataType=sfix(16)  OutScaling=2^0
  Mux : Mux  Inputs=3
  S-Function : S-Function  FunctionName=table3v5  Parameters=x,y,z,tab  EnableBusSupport=off
  Interp Value : Outport  OutDataType=sfix(16)  OutScaling=2^0
  wires:
  S-Function/1 -> Interp Value/1
  Mux/1 -> S-Function/1
  X/1 -> Mux/1
  Y/1 -> Mux/2
  Z/1 -> Mux/3

== system gtm_aeromodel/get aero forces and moments/AERODYNAMICS/Force  Coefficients/LIFT/CLQWB/clqwb_ ==
  Z : Inport  OutDataType=sfix(16)  OutScaling=2^0
  S-Function : S-Function  FunctionName=table1v5  Parameters=z,tab  EnableBusSupport=off
  Interp Value : Outport  OutDataType=sfix(16)  OutScaling=2^0
  wires:
  S-Function/1 -> Interp Value/1
  Z/1 -> S-Function/1

== system gtm_aeromodel/get aero forces and moments/AERODYNAMICS/Force  Coefficients/LIFT/CLQWB/clqwbfr ==
  altitude : Inport  OutDataType=sfix(16)  OutScaling=2^0
  mach1 : Inport  Port=2  OutDataType=sfix(16)  OutScaling=2^0
  Enable : EnablePort
  clqwbfr_ : Subsystem  mask(2-D Table){y=clqwbfrx_FHP, z=clqwbfry_FMACH, tab=clqwbfr}
      mask prompts: y "Y vector:"; z "Z vector:"; tab "Table:"
      mask help: 2-D Table Look Up. Enter monotonic Y and Z vectors and a matrix of 2-D tables. See the help for more info.
      mask Help: The Y and Z vectors must be monotonic.  Y  indexes into the columns of the 2-D table & Z indexes into the rows of the 2-D tables.   The input values are y and z respectively (e.g., top port = y).
      mask Display: plot(-10,-10,110,110,[90,50,10],[90,40,30],[90,50,10],[50,26,20],[90,50,10],[22,13,10])
  clqwbfr : Outport  OutDataType=sfix(16)  OutScaling=2^0  InitialOutput=0
  wires:
  clqwbfr_/1(Interp Value) -> clqwbfr/1
  mach1/1 -> clqwbfr_/2(Z)
  altitude/1 -> clqwbfr_/1(Y)

== system gtm_aeromodel/get aero forces and moments/AERODYNAMICS/Force  Coefficients/LIFT/CLSPOIL/cl_sp_int ==
  flap : Inport  OutDataType=sfix(16)  OutScaling=2^0
  alpha : Inport  Port=2  OutDataType=sfix(16)  OutScaling=2^0
  dsl : Inport  Port=3  OutDataType=sfix(16)  OutScaling=2^0
  dsb : Inport  Port=4  OutDataType=sfix(16)  OutScaling=2^0
  dsr : Inport  Port=5  OutDataType=sfix(16)  OutScaling=2^0
  Enable : EnablePort
  Sum : Sum  Inputs=+-  OutDataType=sfix(16)  OutScaling=2^0  SaturateOnIntegerOverflow=on  InputSameDT=on  OutDataTypeStr=Inherit: Same as first input
  Sum1 : Sum  Inputs=-+  OutDataType=sfix(16)  OutScaling=2^0  SaturateOnIntegerOverflow=on  InputSameDT=on  OutDataTypeStr=Inherit: Same as first input
  Sum2 : Sum  OutDataType=sfix(16)  OutScaling=2^0  SaturateOnIntegerOverflow=on  InputSameDT=on  OutDataTypeStr=Inherit: Same as first input
  dclwbdsbp : Subsystem  mask(1-2-3 Table){@1=dclwbdsldfx_DSL, @2=dclwbdsldfy_FALPHA, @3=dclwbdsldfz_FLPDEF, @4=dclwbdsldf}
      mask prompts: @1 "X vector:"; @2 "Y vector:"; @3 "Z vector:"; @4 "Table:"
      mask help: 3-D Table Look Up. Enter monotonic X, Y and Z vectors and a matrix of 2-D tables. See the help for more info.
      mask init:
      | x=@1;y=@2;z=@3;tab=@4;
      mask Help: The X, Y and Z vectors must be monotonic.   The 3-D table is a horizontal concatenation of  2-D tables.  X  indexes into the columns of the 2-D tables & Y indexes into the rows of the 2-D tables.  Z indexes into the table levels (starting with the 1st 2-D table).   The input values are x, y and z respectively (e.g., top port = x).
      mask Display: plot([0 2 2 0 0],[0 0 2 2 0],[0 2 2.9 0.95 0],[2 2 2.7 2.7 2],[2 2.9 2.9 2 2],[0 0.85 2.7 2 0])
  dclwbdsldf : Subsystem  mask(1-2-3 Table){@1=dclwbdsldfx_DSL, @2=dclwbdsldfy_FALPHA, @3=dclwbdsldfz_FLPDEF, @4=dclwbdsldf}
      mask prompts: @1 "X vector:"; @2 "Y vector:"; @3 "Z vector:"; @4 "Table:"
      mask help: 3-D Table Look Up. Enter monotonic X, Y and Z vectors and a matrix of 2-D tables. See the help for more info.
      mask init:
      | x=@1;y=@2;z=@3;tab=@4;
      mask Help: The X, Y and Z vectors must be monotonic.   The 3-D table is a horizontal concatenation of  2-D tables.  X  indexes into the columns of the 2-D tables & Y indexes into the rows of the 2-D tables.  Z indexes into the table levels (starting with the 1st 2-D table).   The input values are x, y and z respectively (e.g., top port = x).
      mask Display: plot([0 2 2 0 0],[0 0 2 2 0],[0 2 2.9 0.95 0],[2 2 2.7 2.7 2],[2 2.9 2.9 2 2],[0 0.85 2.7 2 0])
  dclwbdsldf1 : Subsystem  mask(1-2-3 Table){@1=dclwbdsldfx_DSL, @2=dclwbdsldfy_FALPHA, @3=dclwbdsldfz_FLPDEF, @4=dclwbdsldf}
      mask prompts: @1 "X vector:"; @2 "Y vector:"; @3 "Z vector:"; @4 "Table:"
      mask help: 3-D Table Look Up. Enter monotonic X, Y and Z vectors and a matrix of 2-D tables. See the help for more info.
      mask init:
      | x=@1;y=@2;z=@3;tab=@4;
      mask Help: The X, Y and Z vectors must be monotonic.   The 3-D table is a horizontal concatenation of  2-D tables.  X  indexes into the columns of the 2-D tables & Y indexes into the rows of the 2-D tables.  Z indexes into the table levels (starting with the 1st 2-D table).   The input values are x, y and z respectively (e.g., top port = x).
      mask Display: plot([0 2 2 0 0],[0 0 2 2 0],[0 2 2.9 0.95 0],[2 2 2.7 2.7 2],[2 2.9 2.9 2 2],[0 0.85 2.7 2 0])
  cl_sp_int : Outport  OutDataType=sfix(16)  OutScaling=2^0  InitialOutput=0
  wires:
  Sum1/1 -> Sum2/2
  Sum/1 -> Sum2/1
  Sum2/1 -> cl_sp_int/1
  dclwbdsbp/1(Interp Value) -> Sum1/1, Sum/2
  dclwbdsldf1/1(Interp Value) -> Sum1/2
  flap/1 -> dclwbdsldf/3(Z), dclwbdsbp/3(Z), dclwbdsldf1/3(Z)
  dclwbdsldf/1(Interp Value) -> Sum/1
  alpha/1 -> dclwbdsldf/2(Y), dclwbdsbp/2(Y), dclwbdsldf1/2(Y)
  dsl/1 -> dclwbdsldf/1(X)
  dsr/1 -> dclwbdsldf1/1(X)
  dsb/1 -> dclwbdsbp/1(X)

== system gtm_aeromodel/get aero forces and moments/AERODYNAMICS/Force  Coefficients/LIFT/CLSPOIL/dcldsbfr ==
  flex : Inport  OutDataType=sfix(16)  OutScaling=2^0
  altitude : Inport  Port=2  OutDataType=sfix(16)  OutScaling=2^0
  mach : Inport  Port=3  OutDataType=sfix(16)  OutScaling=2^0
  Switch7 : Switch  Threshold=0.5  SaturateOnIntegerOverflow=on  InputSameDT=on
  dcldsbfr_ : Subsystem  mask(2-D Table){y=dcldsbfrx_FHP, z=dcldsbfry_FMACH, tab=dcldsbfr}
      mask prompts: y "Y vector:"; z "Z vector:"; tab "Table:"
      mask help: 2-D Table Look Up. Enter monotonic Y and Z vectors and a matrix of 2-D tables. See the help for more info.
      mask Help: The Y and Z vectors must be monotonic.  Y  indexes into the columns of the 2-D table & Z indexes into the rows of the 2-D tables.   The input values are y and z respectively (e.g., top port = y).
      mask Display: plot(-10,-10,110,110,[90,50,10],[90,40,30],[90,50,10],[50,26,20],[90,50,10],[22,13,10])
  one : Constant  OutDataType=sfix(16)  OutScaling=2^0
  dcldsbfr : Outport  OutDataType=sfix(16)  OutScaling=2^0  InitialOutput=0
  wires:
  Switch7/1 -> dcldsbfr/1
  dcldsbfr_/1(Interp Value) -> Switch7/1
  one/1 -> Switch7/3
  flex/1 -> Switch7/2
  mach/1 -> dcldsbfr_/2(Z)
  altitude/1 -> dcldsbfr_/1(Y)

== system gtm_aeromodel/get aero forces and moments/AERODYNAMICS/Force  Coefficients/LIFT/CLSPOIL/dclwbdsb ==
  X : Inport  OutDataType=sfix(16)  OutScaling=2^0
  Y : Inport  Port=2  OutDataType=sfix(16)  OutScaling=2^0
  Z : Inport  Port=3  OutDataType=sfix(16)  OutScaling=2^0
  Mux : Mux  Inputs=3
  S-Function : S-Function  FunctionName=table3v5  Parameters=x,y,z,tab  EnableBusSupport=off
  Interp Value : Outport  OutDataType=sfix(16)  OutScaling=2^0
  wires:
  Z/1 -> Mux/3
  Y/1 -> Mux/2
  X/1 -> Mux/1
  Mux/1 -> S-Function/1
  S-Function/1 -> Interp Value/1

== system gtm_aeromodel/get aero forces and moments/AERODYNAMICS/Force  Coefficients/LIFT/CLSPOIL/dclwbdsb_ ==
  X : Inport  OutDataType=sfix(16)  OutScaling=2^0
  Y : Inport  Port=2  OutDataType=sfix(16)  OutScaling=2^0
  Z : Inport  Port=3  OutDataType=sfix(16)  OutScaling=2^0
  Mux : Mux  Inputs=3
  S-Function : S-Function  FunctionName=table3v5  Parameters=x,y,z,tab  EnableBusSupport=off
  Interp Value : Outport  OutDataType=sfix(16)  OutScaling=2^0
  wires:
  S-Function/1 -> Interp Value/1
  Mux/1 -> S-Function/1
  X/1 -> Mux/1
  Y/1 -> Mux/2
  Z/1 -> Mux/3

== system gtm_aeromodel/get aero forces and moments/AERODYNAMICS/Force  Coefficients/LIFT/CLSPOIL/dclwbdsl ==
  X : Inport  OutDataType=sfix(16)  OutScaling=2^0
  Y : Inport  Port=2  OutDataType=sfix(16)  OutScaling=2^0
  Z : Inport  Port=3  OutDataType=sfix(16)  OutScaling=2^0
  Mux : Mux  Inputs=3
  S-Function : S-Function  FunctionName=table3v5  Parameters=x,y,z,tab  EnableBusSupport=off
  Interp Value : Outport  OutDataType=sfix(16)  OutScaling=2^0
  wires:
  Z/1 -> Mux/3
  Y/1 -> Mux/2
  X/1 -> Mux/1
  Mux/1 -> S-Function/1
  S-Function/1 -> Interp Value/1

== system gtm_aeromodel/get aero forces and moments/AERODYNAMICS/Force  Coefficients/LIFT/CLSPOIL/dclwbdsl1 ==
  X : Inport  OutDataType=sfix(16)  OutScaling=2^0
  Y : Inport  Port=2  OutDataType=sfix(16)  OutScaling=2^0
  Z : Inport  Port=3  OutDataType=sfix(16)  OutScaling=2^0
  Mux : Mux  Inputs=3
  S-Function : S-Function  FunctionName=table3v5  Parameters=x,y,z,tab  EnableBusSupport=off
  Interp Value : Outport  OutDataType=sfix(16)  OutScaling=2^0
  wires:
  S-Function/1 -> Interp Value/1
  Mux/1 -> S-Function/1
  X/1 -> Mux/1
  Y/1 -> Mux/2
  Z/1 -> Mux/3

== system gtm_aeromodel/get aero forces and moments/AERODYNAMICS/Force  Coefficients/LIFT/CLSPOIL/dclwbdsl_ ==
  X : Inport  OutDataType=sfix(16)  OutScaling=2^0
  Y : Inport  Port=2  OutDataType=sfix(16)  OutScaling=2^0
  Z : Inport  Port=3  OutDataType=sfix(16)  OutScaling=2^0
  Mux : Mux  Inputs=3
  S-Function : S-Function  FunctionName=table3v5  Parameters=x,y,z,tab  EnableBusSupport=off
  Interp Value : Outport  OutDataType=sfix(16)  OutScaling=2^0
  wires:
  S-Function/1 -> Interp Value/1
  Mux/1 -> S-Function/1
  X/1 -> Mux/1
  Y/1 -> Mux/2
  Z/1 -> Mux/3

== system gtm_aeromodel/get aero forces and moments/AERODYNAMICS/Force  Coefficients/LIFT/CLSPOIL/dclwbdsl_1 ==
  X : Inport  OutDataType=sfix(16)  OutScaling=2^0
  Y : Inport  Port=2  OutDataType=sfix(16)  OutScaling=2^0
  Z : Inport  Port=3  OutDataType=sfix(16)  OutScaling=2^0
  Mux : Mux  Inputs=3
  S-Function : S-Function  FunctionName=table3v5  Parameters=x,y,z,tab  EnableBusSupport=off
  Interp Value : Outport  OutDataType=sfix(16)  OutScaling=2^0
  wires:
  Z/1 -> Mux/3
  Y/1 -> Mux/2
  X/1 -> Mux/1
  Mux/1 -> S-Function/1
  S-Function/1 -> Interp Value/1

== system gtm_aeromodel/get aero forces and moments/AERODYNAMICS/Force  Coefficients/LIFT/CLSPOIL/dclwbdsl_2 ==
  X : Inport  OutDataType=sfix(16)  OutScaling=2^0
  Y : Inport  Port=2  OutDataType=sfix(16)  OutScaling=2^0
  Z : Inport  Port=3  OutDataType=sfix(16)  OutScaling=2^0
  Mux : Mux  Inputs=3
  S-Function : S-Function  FunctionName=table3v5  Parameters=x,y,z,tab  EnableBusSupport=off
  Interp Value : Outport  OutDataType=sfix(16)  OutScaling=2^0
  wires:
  S-Function/1 -> Interp Value/1
  Mux/1 -> S-Function/1
  X/1 -> Mux/1
  Y/1 -> Mux/2
  Z/1 -> Mux/3

== system gtm_aeromodel/get aero forces and moments/AERODYNAMICS/Force  Coefficients/LIFT/CLSPOIL/dclwbdsl_3 ==
  X : Inport  OutDataType=sfix(16)  OutScaling=2^0
  Y : Inport  Port=2  OutDataType=sfix(16)  OutScaling=2^0
  Z : Inport  Port=3  OutDataType=sfix(16)  OutScaling=2^0
  Mux : Mux  Inputs=3
  S-Function : S-Function  FunctionName=table3v5  Parameters=x,y,z,tab  EnableBusSupport=off
  Interp Value : Outport  OutDataType=sfix(16)  OutScaling=2^0
  wires:
  Z/1 -> Mux/3
  Y/1 -> Mux/2
  X/1 -> Mux/1
  Mux/1 -> S-Function/1
  S-Function/1 -> Interp Value/1

== system gtm_aeromodel/get aero forces and moments/AERODYNAMICS/Force  Coefficients/LIFT/CLTP/clat ==
  Z : Inport  OutDataType=sfix(16)  OutScaling=2^0
  S-Function : S-Function  FunctionName=table1v5  Parameters=z,tab  EnableBusSupport=off
  Interp Value : Outport  OutDataType=sfix(16)  OutScaling=2^0
  wires:
  S-Function/1 -> Interp Value/1
  Z/1 -> S-Function/1

== system gtm_aeromodel/get aero forces and moments/AERODYNAMICS/Force  Coefficients/LIFT/CLTP/cltailflx ==
  note: tddco2g=fqadot*fcbar/(2*32.174)
  altitude : Inport  OutDataType=sfix(16)  OutScaling=2^0
  Mach : Inport  Port=2  OutDataType=sfix(16)  OutScaling=2^0
  norm acc g's : Inport  Port=3  OutDataType=sfix(16)  OutScaling=2^0
  qdot : Inport  Port=4  OutDataType=sfix(16)  OutScaling=2^0
  Enable : EnablePort
  Fcn1 : Fcn  Expr=1/u
  Product1 : Product  OutDataType=sfix(16)  OutScaling=2^0  SaturateOnIntegerOverflow=on  RndMeth=Zero  InputSameDT=on  OutDataTypeStr=Inherit: Same as first input
  Product2 : Product  Inputs=3  OutDataType=sfix(16)  OutScaling=2^0  SaturateOnIntegerOverflow=on  RndMeth=Zero  InputSameDT=on  OutDataTypeStr=Inherit: Same as first input
  Product3 : Product  OutDataType=sfix(16)  OutScaling=2^0  SaturateOnIntegerOverflow=on  RndMeth=Zero  InputSameDT=on  OutDataTypeStr=Inherit: Same as first input
  Product4 : Product  OutDataType=sfix(16)  OutScaling=2^0  SaturateOnIntegerOverflow=on  RndMeth=Zero  InputSameDT=on  OutDataTypeStr=Inherit: Same as first input
  Sum2 : Sum  OutDataType=sfix(16)  OutScaling=2^0  SaturateOnIntegerOverflow=on  InputSameDT=on  OutDataTypeStr=Inherit: Same as first input
  Wing Chord : Constant  Value=A_CW  OutDataType=sfix(16)  OutScaling=2^0
  Wing Chord1 : Constant  Value=2  OutDataType=sfix(16)  OutScaling=2^0
  Wing Chord2 : Constant  Value=constants.g  OutDataType=sfix(16)  OutScaling=2^0
  clatfr_ : Subsystem  mask(2-D Table){y=clatfrx_FHP, z=clatfry_FMACH, tab=clatfr}
      mask prompts: y "Y vector:"; z "Z vector:"; tab "Table:"
      mask help: 2-D Table Look Up. Enter monotonic Y and Z vectors and a matrix of 2-D tables. See the help for more info.
      mask Help: The Y and Z vectors must be monotonic.  Y  indexes into the columns of the 2-D table & Z indexes into the rows of the 2-D tables.   The input values are y and z respectively (e.g., top port = y).
      mask Display: plot(-10,-10,110,110,[90,50,10],[90,40,30],[90,50,10],[50,26,20],[90,50,10],[22,13,10])
  cltdd : Subsystem  mask(2-D Table){y=cltddx_FHP, z=cltddy_FMACH, tab=cltdd}
      mask prompts: y "Y vector:"; z "Z vector:"; tab "Table:"
      mask help: 2-D Table Look Up. Enter monotonic Y and Z vectors and a matrix of 2-D tables. See the help for more info.
      mask Help: The Y and Z vectors must be monotonic.  Y  indexes into the columns of the 2-D table & Z indexes into the rows of the 2-D tables.   The input values are y and z respectively (e.g., top port = y).
      mask Display: plot(-10,-10,110,110,[90,50,10],[90,40,30],[90,50,10],[50,26,20],[90,50,10],[22,13,10])
  clzdd : Subsystem  mask(2-D Table){y=clzddx_FHP, z=clzddy_FMACH, tab=clzdd}
      mask prompts: y "Y vector:"; z "Z vector:"; tab "Table:"
      mask help: 2-D Table Look Up. Enter monotonic Y and Z vectors and a matrix of 2-D tables. See the help for more info.
      mask Help: The Y and Z vectors must be monotonic.  Y  indexes into the columns of the 2-D table & Z indexes into the rows of the 2-D tables.   The input values are y and z respectively (e.g., top port = y).
      mask Display: plot(-10,-10,110,110,[90,50,10],[90,40,30],[90,50,10],[50,26,20],[90,50,10],[22,13,10])
  cltflx : Outport  OutDataType=sfix(16)  OutScaling=2^0  InitialOutput=0
  clatfr : Outport  Port=2  OutDataType=sfix(16)  OutScaling=2^0  InitialOutput=0
  wires:
  Wing Chord1/1 -> Product4/1
  Fcn1/1 -> Product2/3
  Product4/1 -> Fcn1/1
  Wing Chord2/1 -> Product4/2
  clatfr_/1(Interp Value) -> clatfr/1
  altitude/1 -> clatfr_/1(Y), cltdd/1(Y), clzdd/1(Y)
  Product3/1 -> Product2/2
  qdot/1 -> Product3/1
  Wing Chord/1 -> Product3/2
  Product2/1 -> Sum2/2
  Product1/1 -> Sum2/1
  Mach/1 -> clatfr_/2(Z), clzdd/2(Z), cltdd/2(Z)
  cltdd/1(Interp Value) -> Product2/1
  clzdd/1(Interp Value) -> Product1/1
  norm acc g's/1 -> Product1/2
  Sum2/1 -> cltflx/1
